simulink model "chaser_target_slosh"  (R2024a)
settings: Solver=VariableStepAuto  StartTime=0.0  StopTime=10.0  RelTol=1e-3
values from neighbouring files (symbols this model uses):
  dispslosh = 0.2    [main.m]
undefined symbols (not defined in the file or in its folder): chaser, InvDyn, KIN, reaction_wheels, slosh, solar_panel_big_reduced_FEM, solar_panel_target_reduced_FEM, target, ureal, uss, wn_big, wn_target
libraries: RCTblocks x54, SDTlibV1 x44
(part 3 of 3)

== system chaser_target_slosh/Solar panels//Sloshing/sloshing1/zaxis4 ==
  Xddot : Inport  PortDimensions=6
  2*xi : RCTblocks/Uncertain State Space  Tag=USS  USystem=uss(xi)*eye(3)  UValue=[]  X0=[]  uX0=[]
  Add1 : Sum
  Add2 : Sum
  Add3 : Sum  Inputs=--
  Demux : Demux  Outputs=[3 3]
  Ground : Ground
  Integrator : Integrator  InitialCondition=[0;0;0]
  Integrator1 : Integrator  InitialCondition=[0;0;0]
  Mux1 : Mux  Inputs=[3 3]
  Terminator : Terminator
  m1 : RCTblocks/Uncertain State Space  Tag=USS  USystem=1/uss(m1)*eye(3)  UValue=[]  X0=[]  uX0=[]
  "omega1 " : RCTblocks/Uncertain State Space  Tag=USS  USystem=uss(w1)*eye(3)  UValue=[]  X0=[]  uX0=[]
  W_body/. : Outport  PortDimensions=6  VectorParamsAs1DForOutWhenUnconnected=off
  wires:
  "omega1 "/1 -> Add1/1
  Integrator/1 -> 2*xi/1, Integrator1/1  "x dot"
  Integrator1/1 -> "omega1 "/1  "x"
  2*xi/1 -> Add1/2
  Mux1/1 -> W_body/./1
  Ground/1 -> Mux1/2
  Xddot/1 -> Demux/1  "[ Xddot(P) ]/Rb"
  Demux/2 -> Terminator/1
  Add3/1 -> Integrator/1  "x dot dot"
  Add1/1 -> Add2/1, Mux1/1
  Demux/1 -> Add3/1
  m1/1 -> Add3/2
  Add2/1 -> m1/1

== system chaser_target_slosh/Solar panels//Sloshing/sloshing1/zaxis5 ==
  Xddot : Inport  PortDimensions=6
  2*xi : RCTblocks/Uncertain State Space  Tag=USS  USystem=uss(xi)*eye(3)  UValue=[]  X0=[]  uX0=[]
  Add1 : Sum
  Add2 : Sum
  Add3 : Sum  Inputs=--
  Demux : Demux  Outputs=[3 3]
  Ground : Ground
  Integrator : Integrator  InitialCondition=[0;0;0]
  Integrator1 : Integrator  InitialCondition=[0;0;0]
  Mux1 : Mux  Inputs=[3 3]
  Terminator : Terminator
  m1 : RCTblocks/Uncertain State Space  Tag=USS  USystem=1/uss(m1)*eye(3)  UValue=[]  X0=[]  uX0=[]
  "omega1 " : RCTblocks/Uncertain State Space  Tag=USS  USystem=uss(w1)*eye(3)  UValue=[]  X0=[]  uX0=[]
  W_body/. : Outport  PortDimensions=6  VectorParamsAs1DForOutWhenUnconnected=off
  wires:
  "omega1 "/1 -> Add1/1
  Integrator/1 -> 2*xi/1, Integrator1/1  "x dot"
  Integrator1/1 -> "omega1 "/1  "x"
  2*xi/1 -> Add1/2
  Mux1/1 -> W_body/./1
  Ground/1 -> Mux1/2
  Xddot/1 -> Demux/1  "[ Xddot(P) ]/Rb"
  Demux/2 -> Terminator/1
  Add3/1 -> Integrator/1  "x dot dot"
  Add1/1 -> Add2/1, Mux1/1
  Demux/1 -> Add3/1
  m1/1 -> Add3/2
  Add2/1 -> m1/1

== system chaser_target_slosh/Solar panels//Sloshing/sloshing1/zaxis6 ==
  Xddot : Inport  PortDimensions=6
  2*xi : RCTblocks/Uncertain State Space  Tag=USS  USystem=uss(xi)*eye(3)  UValue=[]  X0=[]  uX0=[]
  Add1 : Sum
  Add2 : Sum
  Add3 : Sum  Inputs=--
  Demux : Demux  Outputs=[3 3]
  Ground : Ground
  Integrator : Integrator  InitialCondition=[0;0;0]
  Integrator1 : Integrator  InitialCondition=[0;0;0]
  Mux1 : Mux  Inputs=[3 3]
  Terminator : Terminator
  m1 : RCTblocks/Uncertain State Space  Tag=USS  USystem=1/uss(m1)*eye(3)  UValue=[]  X0=[]  uX0=[]
  "omega1 " : RCTblocks/Uncertain State Space  Tag=USS  USystem=uss(w1)*eye(3)  UValue=[]  X0=[]  uX0=[]
  W_body/. : Outport  PortDimensions=6  VectorParamsAs1DForOutWhenUnconnected=off
  wires:
  "omega1 "/1 -> Add1/1
  Integrator/1 -> 2*xi/1, Integrator1/1  "x dot"
  Integrator1/1 -> "omega1 "/1  "x"
  2*xi/1 -> Add1/2
  Mux1/1 -> W_body/./1
  Ground/1 -> Mux1/2
  Xddot/1 -> Demux/1  "[ Xddot(P) ]/Rb"
  Demux/2 -> Terminator/1
  Add3/1 -> Integrator/1  "x dot dot"
  Add1/1 -> Add2/1, Mux1/1
  Demux/1 -> Add3/1
  m1/1 -> Add3/2
  Add2/1 -> m1/1
